simulink model "RobotSystem_2"  (Simulink 5.0)
settings: Solver=ode45  StartTime=0.0  StopTime=SimulationTime  RelTol=1e-3
values from neighbouring files (symbols this model uses):
  d1 = d1 * d1_err    [MakeFourMassRobot.m]
  d2 = d2 * d2_err    [MakeFourMassRobot.m]
  d3 = d3 * d3_err    [MakeFourMassRobot.m]
  DelayTime = DelayTime * DelayTime_err    [MakeFourMassRobot.m]
  fa1 = fa1 * fa1_err    [MakeFourMassRobot.m]
  fa2 = fa2 * fa2_err    [MakeFourMassRobot.m]
  fa3 = fa3 * fa3_err    [MakeFourMassRobot.m]
  FF = 0.50    (= 0.5)    [Controller_1.m]
  fm = fm * fm_err    [MakeFourMassRobot.m]
  Gain = Gain * Gain_err    [MakeFourMassRobot.m]
  gear_ratio = 220    [MakeFourMassRobot.m]
  Ja1 = Ja1 * Ja1_err    [MakeFourMassRobot.m]
  Ja2 = Ja2 * Ja2_err    [MakeFourMassRobot.m]
  Ja3 = Ja3 * Ja3_err    [MakeFourMassRobot.m]
  Jm = Jm * Jm_err    [MakeFourMassRobot.m]
  k1 = k1 * k1_err    [MakeFourMassRobot.m]
  k1_low = k1_low * k1_low_err    [MakeFourMassRobot.m]
  k1_low_pos = 0    [MakeFourMassRobot.m]
  k1_pos = k1_pos * k1_pos_err    [MakeFourMassRobot.m]
  k2 = k2 * k2_err    [MakeFourMassRobot.m]
  k3 = k3 * k3_err    [MakeFourMassRobot.m]
  KD = 1.2    [Controller_1.m]
  KI = 30    [Controller_1.m]
  KP = 12    [Controller_1.m]
  len1 = 20    [MakeFourMassRobot.m]
  len2 = 600    [MakeFourMassRobot.m]
  len3 = 1530    [MakeFourMassRobot.m]
  MotorDisturbance1 = 3.5    [SetParameters.m]
  MotorDisturbance2 = 3.5    [SetParameters.m]
  MotorDisturbance3 = 7    [SetParameters.m]
  MotorDisturbance4 = 4.5    [SetParameters.m]
  MotorDisturbanceChirpAmplitude1 = 1.5    [SetParameters.m]
  MotorDisturbanceChirpAmplitude2 = 1.5    [SetParameters.m]
  MotorDisturbanceChirpEndFrequency1 = 2    [SetParameters.m]
  MotorDisturbanceChirpEndFrequency2 = 2    [SetParameters.m]
  MotorDisturbanceChirpEndTime1 = 21.5    [SetParameters.m]
  MotorDisturbanceChirpEndTime2 = 48    [SetParameters.m]
  MotorDisturbanceChirpStartFrequency1 = 15    [SetParameters.m]
  MotorDisturbanceChirpStartFrequency2 = 15    [SetParameters.m]
  MotorDisturbanceChirpStartTime1 = 16.5    [SetParameters.m]
  MotorDisturbanceChirpStartTime2 = 43    [SetParameters.m]
  MotorDisturbanceOff1 = 5.5    [SetParameters.m]
  MotorDisturbanceOff2 = 25    [SetParameters.m]
  MotorDisturbanceOff3 = 1000    [SetParameters.m]
  MotorDisturbanceOff4 = 32.5    [SetParameters.m]
  MotorDisturbanceOn1 = 5    [SetParameters.m]
  MotorDisturbanceOn2 = 6    [SetParameters.m]
  MotorDisturbanceOn3 = 25    [SetParameters.m]
  MotorDisturbanceOn4 = 32    [SetParameters.m]
  NoiseP = 0.5E-10    (= 5e-11)    [SetParameters.m]
  NoiseTs = 0.5E-3    (= 0.0005)    [SetParameters.m]
  SampleTime = 0.5E-3    (= 0.0005)    [SetParameters.m]
  SimulationTime = 55    [SetParameters.m]
  ToolDisturbance1 = 5    [SetParameters.m]
  ToolDisturbance2 = -7    [SetParameters.m]
  ToolDisturbance3 = 5    [SetParameters.m]
  ToolDisturbanceChirpAmplitude1 = 1.5    [SetParameters.m]
  ToolDisturbanceChirpAmplitude2 = 1.5    [SetParameters.m]
  ToolDisturbanceChirpEndFrequency1 = 2    [SetParameters.m]
  ToolDisturbanceChirpEndFrequency2 = 2    [SetParameters.m]
  ToolDisturbanceChirpEndTime1 = 15.5    [SetParameters.m]
  ToolDisturbanceChirpEndTime2 = 42    [SetParameters.m]
  ToolDisturbanceChirpStartFrequency1 = 15    [SetParameters.m]
  ToolDisturbanceChirpStartFrequency2 = 15    [SetParameters.m]
  ToolDisturbanceChirpStartTime1 = 10.5    [SetParameters.m]
  ToolDisturbanceChirpStartTime2 = 37    [SetParameters.m]
  ToolDisturbanceOff1 = 0.5    [SetParameters.m]
  ToolDisturbanceOff2 = 1000    [SetParameters.m]
  ToolDisturbanceOff3 = 27.5    [SetParameters.m]
  ToolDisturbanceOn1 = 0    [SetParameters.m]
  ToolDisturbanceOn2 = 25    [SetParameters.m]
  ToolDisturbanceOn3 = 27    [SetParameters.m]
  TorqueLimitMax = 20    [SetParameters.m]
  TorqueLimitMin = -20    [SetParameters.m]
libraries: simulink x1
settings Model: LastModifiedBy=STMO  ExtModeTrigMode=oneshot  ExtModeArmWhenConnect=off  LimitDataPoints=off  BlockReductionOpt=off  BooleanDataType=off

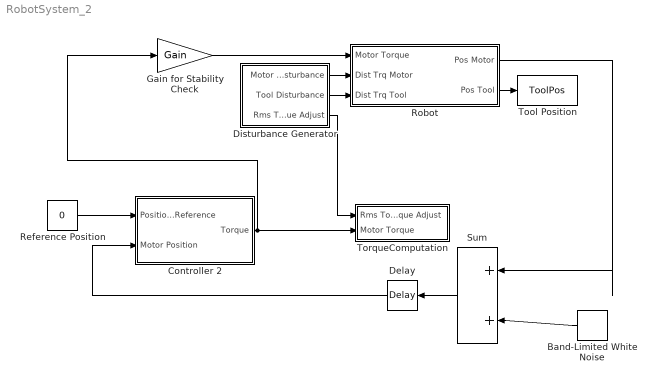
== system RobotSystem_2 ==
  Band-Limited White Noise : simulink/Sources/Band-Limited White Noise  Orientation=left  Cov=[NoiseP]  Ts=NoiseTs  seed=[23341]
  Controller 2 : Subsystem
  Delay : TransportDelay  Orientation=left  DelayTime=DelayTime
  Disturbance Generator : Subsystem
  Gain for Stability Check : Gain  Gain=Gain  SaturateOnIntegerOverflow=on
  Reference Position : Constant  Value=0
  Robot : Subsystem
  Sum : Sum  Orientation=left  Inputs=|++  SaturateOnIntegerOverflow=on
  Tool Position : ToWorkspace  VariableName=ToolPos  SampleTime=-1  SaveFormat=StructureWithTime
  TorqueComputation : Subsystem
  wires:
  Robot/2(Pos Tool) -> Tool Position/1
  Sum/1 -> Delay/1
  Robot/1(Pos Motor) -> Sum/1
  Band-Limited White Noise/1 -> Sum/2
  Disturbance Generator/1(Motor Disturbance) -> Robot/2(Dist Trq Motor)
  Disturbance Generator/2(Tool Disturbance) -> Robot/3(Dist Trq Tool)
  Gain for Stability Check/1 -> Robot/1(Motor Torque)
  Reference Position/1 -> Controller 2/1(Position Reference)
  Delay/1 -> Controller 2/2(Motor Position)
  Controller 2/1(Torque) -> Gain for Stability Check/1, TorqueComputation/2(Motor Torque)
  Disturbance Generator/3(Rms Torque Adjust) -> TorqueComputation/1(Rms Torque Adjust)

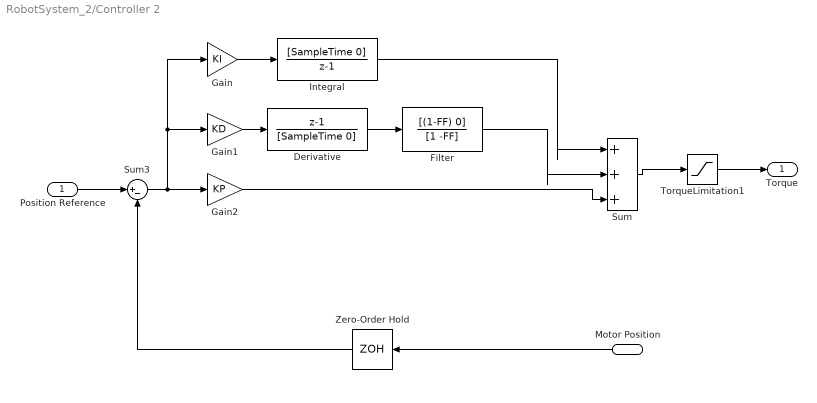
== system RobotSystem_2/Controller 2 ==
  Position Reference : Inport
  Motor Position : Inport  Orientation=left  Port=2
  Derivative : DiscreteTransferFcn  Numerator=[1 -1]  Denominator=[SampleTime 0]  SampleTime=SampleTime
  Filter : DiscreteTransferFcn  Numerator=[(1-FF) 0]  Denominator=[1 -FF]  SampleTime=SampleTime
  Gain : Gain  Gain=KI  SaturateOnIntegerOverflow=on
  Gain1 : Gain  Gain=KD  SaturateOnIntegerOverflow=on
  Gain2 : Gain  Gain=KP  SaturateOnIntegerOverflow=on
  Integral : DiscreteTransferFcn  Numerator=[SampleTime 0]  Denominator=[1 -1]  SampleTime=SampleTime
  Sum : Sum  Inputs=|+++  SaturateOnIntegerOverflow=on
  Sum3 : Sum  Inputs=|+-  SaturateOnIntegerOverflow=on  InputSameDT=on
  TorqueLimitation1 : Saturate  UpperLimit=TorqueLimitMax  LowerLimit=TorqueLimitMin
  Zero-Order Hold : ZeroOrderHold  Orientation=left  SampleTime=SampleTime
  Torque : Outport
  wires:
  Motor Position/1 -> Zero-Order Hold/1
  Position Reference/1 -> Sum3/1
  TorqueLimitation1/1 -> Torque/1
  Zero-Order Hold/1 -> Sum3/2
  Sum/1 -> TorqueLimitation1/1
  Integral/1 -> Sum/1
  Derivative/1 -> Filter/1
  Gain/1 -> Integral/1
  Gain1/1 -> Derivative/1
  Gain2/1 -> Sum/3
  Sum3/1 -> Gain2/1, Gain/1, Gain1/1
  Filter/1 -> Sum/2

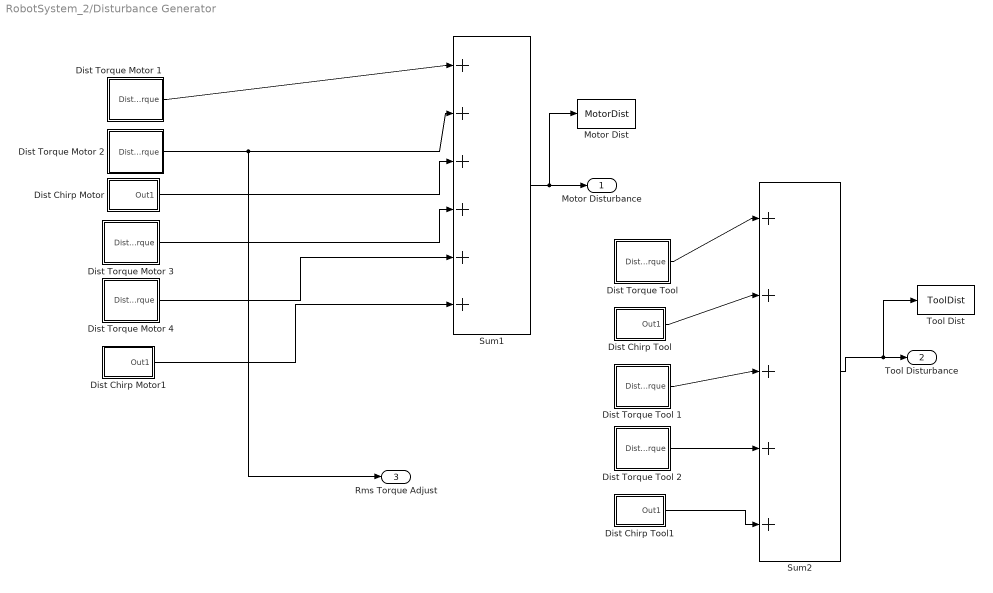
== system RobotSystem_2/Disturbance Generator ==
  Dist Chirp Motor : Subsystem  mask{f1=MotorDisturbanceChirpStartFrequency1, f2=MotorDisturbanceChirpEndFrequency1, T1=MotorDisturbanceChirpStartTime1, T2=MotorDisturbanceChirpEndTime1, Amp=MotorDisturbanceChirpAmplitude1}
      mask prompts: f1 "f1 [Hz]"; f2 "f2 [Hz]"; T1 "T1 [s]"; T2 "T2 [s]"; Amp "Amplitude"
      mask Display: disp('Chirp')
  Dist Chirp Motor1 : Subsystem  mask{f1=MotorDisturbanceChirpStartFrequency2, f2=MotorDisturbanceChirpEndFrequency2, T1=MotorDisturbanceChirpStartTime2, T2=MotorDisturbanceChirpEndTime2, Amp=MotorDisturbanceChirpAmplitude2}
      mask prompts: f1 "f1 [Hz]"; f2 "f2 [Hz]"; T1 "T1 [s]"; T2 "T2 [s]"; Amp "Amplitude"
      mask Display: disp('Chirp')
  Dist Chirp Tool : Subsystem  mask{f1=ToolDisturbanceChirpStartFrequency1, f2=ToolDisturbanceChirpEndFrequency1, T1=ToolDisturbanceChirpStartTime1, T2=ToolDisturbanceChirpEndTime1, Amp=ToolDisturbanceChirpAmplitude1}
      mask prompts: f1 "f1 [Hz]"; f2 "f2 [Hz]"; T1 "T1 [s]"; T2 "T2 [s]"; Amp "Amplitude"
      mask Display: disp('Chirp')
  Dist Chirp Tool1 : Subsystem  mask{f1=ToolDisturbanceChirpStartFrequency2, f2=ToolDisturbanceChirpEndFrequency2, T1=ToolDisturbanceChirpStartTime2, T2=ToolDisturbanceChirpEndTime2, Amp=ToolDisturbanceChirpAmplitude2}
      mask prompts: f1 "f1 [Hz]"; f2 "f2 [Hz]"; T1 "T1 [s]"; T2 "T2 [s]"; Amp "Amplitude"
      mask Display: disp('Chirp')
  Dist Torque Motor 1 : Subsystem  mask{torque=MotorDisturbance1, t1=MotorDisturbanceOn1, t2=MotorDisturbanceOff1}
      mask prompts: torque "Disturbance Torque"; t1 "Pulse On Time"; t2 "Pulse Off Time"
  Dist Torque Motor 2 : Subsystem  mask{torque=MotorDisturbance2, t1=MotorDisturbanceOn2, t2=MotorDisturbanceOff2}
      mask prompts: torque "Disturbance Torque"; t1 "Pulse On Time"; t2 "Pulse Off Time"
  Dist Torque Motor 3 : Subsystem  mask{torque=MotorDisturbance3, t1=MotorDisturbanceOn3, t2=MotorDisturbanceOff3}
      mask prompts: torque "Disturbance Torque"; t1 "Pulse On Time"; t2 "Pulse Off Time"
  Dist Torque Motor 4 : Subsystem  mask{torque=MotorDisturbance4, t1=MotorDisturbanceOn4, t2=MotorDisturbanceOff4}
      mask prompts: torque "Disturbance Torque"; t1 "Pulse On Time"; t2 "Pulse Off Time"
  Dist Torque Tool : Subsystem  mask{torque=ToolDisturbance1, t1=ToolDisturbanceOn1, t2=ToolDisturbanceOff1}
      mask prompts: torque "Disturbance Torque"; t1 "Pulse On Time"; t2 "Pulse Off Time"
  Dist Torque Tool 1 : Subsystem  mask{torque=ToolDisturbance2, t1=ToolDisturbanceOn2, t2=ToolDisturbanceOff2}
      mask prompts: torque "Disturbance Torque"; t1 "Pulse On Time"; t2 "Pulse Off Time"
  Dist Torque Tool 2 : Subsystem  mask{torque=ToolDisturbance3, t1=ToolDisturbanceOn3, t2=ToolDisturbanceOff3}
      mask prompts: torque "Disturbance Torque"; t1 "Pulse On Time"; t2 "Pulse Off Time"
  Motor Dist : ToWorkspace  VariableName=MotorDist  SampleTime=-1  SaveFormat=StructureWithTime
  Sum1 : Sum  Inputs=|++++++  SaturateOnIntegerOverflow=on  InputSameDT=on
  Sum2 : Sum  Inputs=|+++++  SaturateOnIntegerOverflow=on  InputSameDT=on
  Tool Dist : ToWorkspace  VariableName=ToolDist  SampleTime=-1  SaveFormat=StructureWithTime
  Motor Disturbance : Outport
  Tool Disturbance : Outport  Port=2
  Rms Torque Adjust : Outport  Port=3
  wires:
  Dist Torque Motor 1/1(Dist Torque) -> Sum1/1
  Dist Torque Tool/1(Dist Torque) -> Sum2/1
  Dist Chirp Motor/1(Out1) -> Sum1/3
  Dist Chirp Tool/1(Out1) -> Sum2/2
  Sum1/1 -> Motor Dist/1, Motor Disturbance/1
  Sum2/1 -> Tool Disturbance/1, Tool Dist/1
  Dist Torque Motor 3/1(Dist Torque) -> Sum1/4
  Dist Torque Motor 2/1(Dist Torque) -> Sum1/2, Rms Torque Adjust/1
  Dist Torque Tool 1/1(Dist Torque) -> Sum2/3
  Dist Torque Motor 4/1(Dist Torque) -> Sum1/5
  Dist Chirp Motor1/1(Out1) -> Sum1/6
  Dist Chirp Tool1/1(Out1) -> Sum2/5
  Dist Torque Tool 2/1(Dist Torque) -> Sum2/4

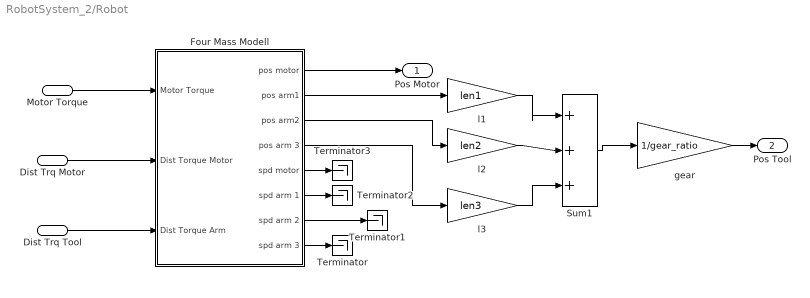
== system RobotSystem_2/Robot ==
  Motor Torque : Inport
  Dist Trq Motor : Inport  Port=2
  Dist Trq Tool : Inport  Port=3
  Four Mass Modell : Subsystem
  Sum1 : Sum  Inputs=|+++  SaturateOnIntegerOverflow=on  InputSameDT=on
  Terminator{,1..3} (4 alike) : Terminator
  gear : Gain  Gain=1/gear_ratio  SaturateOnIntegerOverflow=on
  l1 : Gain  Gain=len1  SaturateOnIntegerOverflow=on
  l2 : Gain  Gain=len2  SaturateOnIntegerOverflow=on
  l3 : Gain  Gain=len3  SaturateOnIntegerOverflow=on
  Pos Motor : Outport
  Pos Tool : Outport  Port=2
  wires:
  Motor Torque/1 -> Four Mass Modell/1(Motor Torque)
  Dist Trq Tool/1 -> Four Mass Modell/3(Dist Torque Arm)
  Dist Trq Motor/1 -> Four Mass Modell/2(Dist Torque Motor)
  Four Mass Modell/1(pos motor) -> Pos Motor/1
  Four Mass Modell/8(spd arm 3) -> Terminator/1
  Four Mass Modell/7(spd arm 2) -> Terminator1/1
  Four Mass Modell/6(spd arm 1) -> Terminator2/1
  Four Mass Modell/5(spd motor) -> Terminator3/1
  Four Mass Modell/3(pos arm2) -> l2/1
  Four Mass Modell/2(pos arm1) -> l1/1
  Four Mass Modell/4(pos arm 3) -> l3/1
  l1/1 -> Sum1/1
  l2/1 -> Sum1/2
  l3/1 -> Sum1/3
  gear/1 -> Pos Tool/1
  Sum1/1 -> gear/1

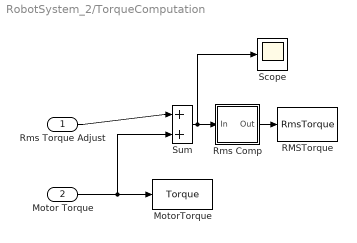
== system RobotSystem_2/TorqueComputation ==
  Rms Torque Adjust : Inport
  Motor Torque : Inport  Port=2
  MotorTorque : ToWorkspace  VariableName=Torque  SampleTime=-1  SaveFormat=StructureWithTime
  RMSTorque : ToWorkspace  VariableName=RmsTorque  SampleTime=-1  SaveFormat=StructureWithTime
  Rms Comp : Subsystem
  Scope : Scope
  Sum : Sum  Inputs=|++  SaturateOnIntegerOverflow=on
  wires:
  Rms Comp/1(Out) -> RMSTorque/1
  Sum/1 -> Rms Comp/1(In), Scope/1
  Rms Torque Adjust/1 -> Sum/1
  Motor Torque/1 -> Sum/2, MotorTorque/1

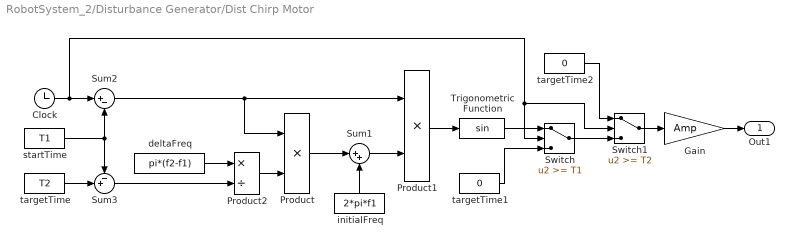
== system RobotSystem_2/Disturbance Generator/Dist Chirp Motor ==
  Clock : Clock
      settings: Decimation=10
  Gain : Gain  Gain=Amp  SaturateOnIntegerOverflow=on
  Product : Product  SaturateOnIntegerOverflow=on  InputSameDT=on
  Product1 : Product  SaturateOnIntegerOverflow=on  InputSameDT=on
  Product2 : Product  Inputs=*/  SaturateOnIntegerOverflow=on  InputSameDT=on
  Sum1 : Sum  Inputs=|++  SaturateOnIntegerOverflow=on  InputSameDT=on
  Sum2 : Sum  Inputs=|+-  SaturateOnIntegerOverflow=on  InputSameDT=on
  Sum3 : Sum  Inputs=-+|  SaturateOnIntegerOverflow=on  InputSameDT=on
  Switch : Switch  Threshold=T1  SaturateOnIntegerOverflow=on  InputSameDT=on
  Switch1 : Switch  Threshold=T2  SaturateOnIntegerOverflow=on  InputSameDT=on
  Trigonometric Function : Trigonometry
  deltaFreq : Constant  Value=pi*(f2-f1)
  initialFreq : Constant  Orientation=up  Value=2*pi*f1
  startTime : Constant  Value=T1
  targetTime : Constant  Value=T2
  targetTime1 : Constant  Value=0
  targetTime2 : Constant  Value=0
  Out1 : Outport
  wires:
  startTime/1 -> Sum3/1, Sum2/2
  Sum2/1 -> Product/1, Product1/1
  Product1/1 -> Trigonometric Function/1
  Sum1/1 -> Product1/2
  Sum3/1 -> Product2/2
  deltaFreq/1 -> Product2/1
  Product2/1 -> Product/2
  targetTime/1 -> Sum3/2
  Clock/1 -> Sum2/1, Switch/2, Switch1/2
  initialFreq/1 -> Sum1/2
  Product/1 -> Sum1/1
  Trigonometric Function/1 -> Switch/1
  targetTime1/1 -> Switch/3
  Switch/1 -> Switch1/3
  Switch1/1 -> Gain/1
  targetTime2/1 -> Switch1/1
  Gain/1 -> Out1/1

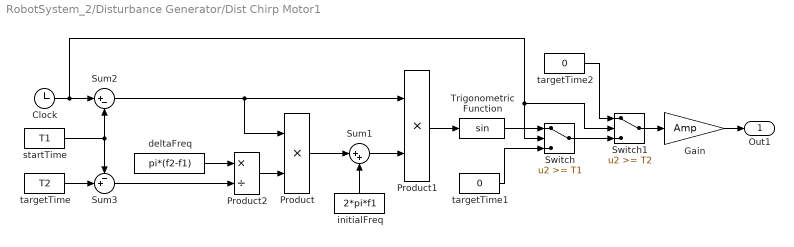
== system RobotSystem_2/Disturbance Generator/Dist Chirp Motor1 ==
  Clock : Clock
      settings: Decimation=10
  Gain : Gain  Gain=Amp  SaturateOnIntegerOverflow=on
  Product : Product  SaturateOnIntegerOverflow=on  InputSameDT=on
  Product1 : Product  SaturateOnIntegerOverflow=on  InputSameDT=on
  Product2 : Product  Inputs=*/  SaturateOnIntegerOverflow=on  InputSameDT=on
  Sum1 : Sum  Inputs=|++  SaturateOnIntegerOverflow=on  InputSameDT=on
  Sum2 : Sum  Inputs=|+-  SaturateOnIntegerOverflow=on  InputSameDT=on
  Sum3 : Sum  Inputs=-+|  SaturateOnIntegerOverflow=on  InputSameDT=on
  Switch : Switch  Threshold=T1  SaturateOnIntegerOverflow=on  InputSameDT=on
  Switch1 : Switch  Threshold=T2  SaturateOnIntegerOverflow=on  InputSameDT=on
  Trigonometric Function : Trigonometry
  deltaFreq : Constant  Value=pi*(f2-f1)
  initialFreq : Constant  Orientation=up  Value=2*pi*f1
  startTime : Constant  Value=T1
  targetTime : Constant  Value=T2
  targetTime1 : Constant  Value=0
  targetTime2 : Constant  Value=0
  Out1 : Outport
  wires:
  startTime/1 -> Sum3/1, Sum2/2
  Sum2/1 -> Product/1, Product1/1
  Product1/1 -> Trigonometric Function/1
  Sum1/1 -> Product1/2
  Sum3/1 -> Product2/2
  deltaFreq/1 -> Product2/1
  Product2/1 -> Product/2
  targetTime/1 -> Sum3/2
  Clock/1 -> Sum2/1, Switch/2, Switch1/2
  initialFreq/1 -> Sum1/2
  Product/1 -> Sum1/1
  Trigonometric Function/1 -> Switch/1
  targetTime1/1 -> Switch/3
  Switch/1 -> Switch1/3
  Switch1/1 -> Gain/1
  targetTime2/1 -> Switch1/1
  Gain/1 -> Out1/1

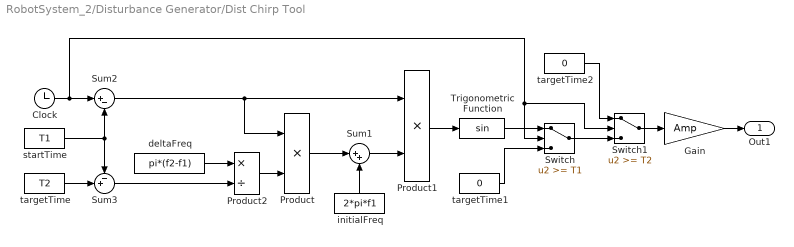
== system RobotSystem_2/Disturbance Generator/Dist Chirp Tool ==
  Clock : Clock
      settings: Decimation=10
  Gain : Gain  Gain=Amp  SaturateOnIntegerOverflow=on
  Product : Product  SaturateOnIntegerOverflow=on  InputSameDT=on
  Product1 : Product  SaturateOnIntegerOverflow=on  InputSameDT=on
  Product2 : Product  Inputs=*/  SaturateOnIntegerOverflow=on  InputSameDT=on
  Sum1 : Sum  Inputs=|++  SaturateOnIntegerOverflow=on  InputSameDT=on
  Sum2 : Sum  Inputs=|+-  SaturateOnIntegerOverflow=on  InputSameDT=on
  Sum3 : Sum  Inputs=-+|  SaturateOnIntegerOverflow=on  InputSameDT=on
  Switch : Switch  Threshold=T1  SaturateOnIntegerOverflow=on  InputSameDT=on
  Switch1 : Switch  Threshold=T2  SaturateOnIntegerOverflow=on  InputSameDT=on
  Trigonometric Function : Trigonometry
  deltaFreq : Constant  Value=pi*(f2-f1)
  initialFreq : Constant  Orientation=up  Value=2*pi*f1
  startTime : Constant  Value=T1
  targetTime : Constant  Value=T2
  targetTime1 : Constant  Value=0
  targetTime2 : Constant  Value=0
  Out1 : Outport
  wires:
  startTime/1 -> Sum3/1, Sum2/2
  Sum2/1 -> Product/1, Product1/1
  Product1/1 -> Trigonometric Function/1
  Sum1/1 -> Product1/2
  Sum3/1 -> Product2/2
  deltaFreq/1 -> Product2/1
  Product2/1 -> Product/2
  targetTime/1 -> Sum3/2
  Clock/1 -> Sum2/1, Switch/2, Switch1/2
  initialFreq/1 -> Sum1/2
  Product/1 -> Sum1/1
  Trigonometric Function/1 -> Switch/1
  targetTime1/1 -> Switch/3
  Switch/1 -> Switch1/3
  Switch1/1 -> Gain/1
  targetTime2/1 -> Switch1/1
  Gain/1 -> Out1/1

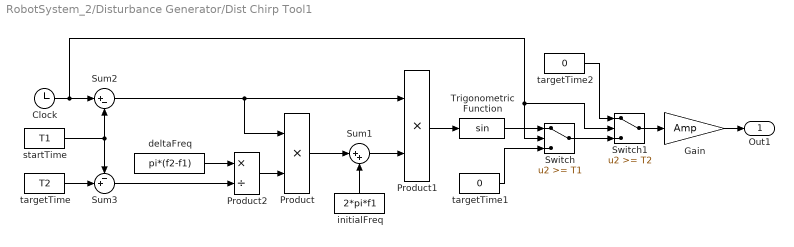
== system RobotSystem_2/Disturbance Generator/Dist Chirp Tool1 ==
  Clock : Clock
      settings: Decimation=10
  Gain : Gain  Gain=Amp  SaturateOnIntegerOverflow=on
  Product : Product  SaturateOnIntegerOverflow=on  InputSameDT=on
  Product1 : Product  SaturateOnIntegerOverflow=on  InputSameDT=on
  Product2 : Product  Inputs=*/  SaturateOnIntegerOverflow=on  InputSameDT=on
  Sum1 : Sum  Inputs=|++  SaturateOnIntegerOverflow=on  InputSameDT=on
  Sum2 : Sum  Inputs=|+-  SaturateOnIntegerOverflow=on  InputSameDT=on
  Sum3 : Sum  Inputs=-+|  SaturateOnIntegerOverflow=on  InputSameDT=on
  Switch : Switch  Threshold=T1  SaturateOnIntegerOverflow=on  InputSameDT=on
  Switch1 : Switch  Threshold=T2  SaturateOnIntegerOverflow=on  InputSameDT=on
  Trigonometric Function : Trigonometry
  deltaFreq : Constant  Value=pi*(f2-f1)
  initialFreq : Constant  Orientation=up  Value=2*pi*f1
  startTime : Constant  Value=T1
  targetTime : Constant  Value=T2
  targetTime1 : Constant  Value=0
  targetTime2 : Constant  Value=0
  Out1 : Outport
  wires:
  startTime/1 -> Sum3/1, Sum2/2
  Sum2/1 -> Product/1, Product1/1
  Product1/1 -> Trigonometric Function/1
  Sum1/1 -> Product1/2
  Sum3/1 -> Product2/2
  deltaFreq/1 -> Product2/1
  Product2/1 -> Product/2
  targetTime/1 -> Sum3/2
  Clock/1 -> Sum2/1, Switch/2, Switch1/2
  initialFreq/1 -> Sum1/2
  Product/1 -> Sum1/1
  Trigonometric Function/1 -> Switch/1
  targetTime1/1 -> Switch/3
  Switch/1 -> Switch1/3
  Switch1/1 -> Gain/1
  targetTime2/1 -> Switch1/1
  Gain/1 -> Out1/1

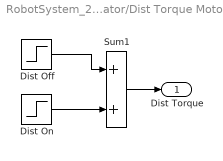
== system RobotSystem_2/Disturbance Generator/Dist Torque Motor 1 ==
  Dist Off : Step  Time=t2  After=-torque  SampleTime=0
  Dist On : Step  Time=t1  After=torque  SampleTime=0
  Sum1 : Sum  Inputs=|++  SaturateOnIntegerOverflow=on  InputSameDT=on
  Dist Torque : Outport
  wires:
  Dist On/1 -> Sum1/2
  Dist Off/1 -> Sum1/1
  Sum1/1 -> Dist Torque/1

== system RobotSystem_2/Disturbance Generator/Dist Torque Motor 2 ==
  Dist Off : Step  Time=t2  After=-torque  SampleTime=0
  Dist On : Step  Time=t1  After=torque  SampleTime=0
  Sum1 : Sum  Inputs=|++  SaturateOnIntegerOverflow=on  InputSameDT=on
  Dist Torque : Outport
  wires:
  Dist On/1 -> Sum1/2
  Dist Off/1 -> Sum1/1
  Sum1/1 -> Dist Torque/1

== system RobotSystem_2/Disturbance Generator/Dist Torque Motor 3 ==
  Dist Off : Step  Time=t2  After=-torque  SampleTime=0
  Dist On : Step  Time=t1  After=torque  SampleTime=0
  Sum1 : Sum  Inputs=|++  SaturateOnIntegerOverflow=on  InputSameDT=on
  Dist Torque : Outport
  wires:
  Dist On/1 -> Sum1/2
  Dist Off/1 -> Sum1/1
  Sum1/1 -> Dist Torque/1

== system RobotSystem_2/Disturbance Generator/Dist Torque Motor 4 ==
  Dist Off : Step  Time=t2  After=-torque  SampleTime=0
  Dist On : Step  Time=t1  After=torque  SampleTime=0
  Sum1 : Sum  Inputs=|++  SaturateOnIntegerOverflow=on  InputSameDT=on
  Dist Torque : Outport
  wires:
  Dist On/1 -> Sum1/2
  Dist Off/1 -> Sum1/1
  Sum1/1 -> Dist Torque/1

== system RobotSystem_2/Disturbance Generator/Dist Torque Tool ==
  Dist Off : Step  Time=t2  After=-torque  SampleTime=0
  Dist On : Step  Time=t1  After=torque  SampleTime=0
  Sum1 : Sum  Inputs=|++  SaturateOnIntegerOverflow=on  InputSameDT=on
  Dist Torque : Outport
  wires:
  Dist On/1 -> Sum1/2
  Dist Off/1 -> Sum1/1
  Sum1/1 -> Dist Torque/1

== system RobotSystem_2/Disturbance Generator/Dist Torque Tool 1 ==
  Dist Off : Step  Time=t2  After=-torque  SampleTime=0
  Dist On : Step  Time=t1  After=torque  SampleTime=0
  Sum1 : Sum  Inputs=|++  SaturateOnIntegerOverflow=on  InputSameDT=on
  Dist Torque : Outport
  wires:
  Dist On/1 -> Sum1/2
  Dist Off/1 -> Sum1/1
  Sum1/1 -> Dist Torque/1

== system RobotSystem_2/Disturbance Generator/Dist Torque Tool 2 ==
  Dist Off : Step  Time=t2  After=-torque  SampleTime=0
  Dist On : Step  Time=t1  After=torque  SampleTime=0
  Sum1 : Sum  Inputs=|++  SaturateOnIntegerOverflow=on  InputSameDT=on
  Dist Torque : Outport
  wires:
  Dist On/1 -> Sum1/2
  Dist Off/1 -> Sum1/1
  Sum1/1 -> Dist Torque/1

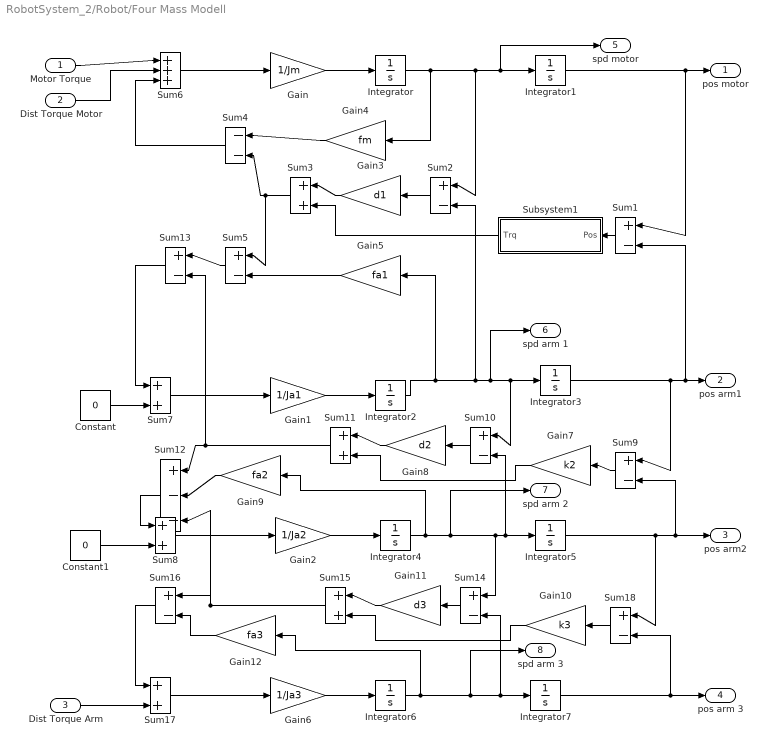
== system RobotSystem_2/Robot/Four Mass Modell ==
  Motor Torque : Inport
  Dist Torque Motor : Inport  Port=2
  Dist Torque Arm : Inport  Port=3
  Constant : Constant  Value=0
  Constant1 : Constant  Value=0
  Gain : Gain  Gain=1/Jm  SaturateOnIntegerOverflow=on
  Gain1 : Gain  Gain=1/Ja1  SaturateOnIntegerOverflow=on
  Gain10 : Gain  Orientation=left  Gain=k3  SaturateOnIntegerOverflow=on
  Gain11 : Gain  Orientation=left  Gain=d3  SaturateOnIntegerOverflow=on
  Gain12 : Gain  Orientation=left  Gain=fa3  SaturateOnIntegerOverflow=on
  Gain2 : Gain  Gain=1/Ja2  SaturateOnIntegerOverflow=on
  Gain3 : Gain  Orientation=left  Gain=d1  SaturateOnIntegerOverflow=on
  Gain4 : Gain  Orientation=left  Gain=fm  SaturateOnIntegerOverflow=on
  Gain5 : Gain  Orientation=left  Gain=fa1  SaturateOnIntegerOverflow=on
  Gain6 : Gain  Gain=1/Ja3  SaturateOnIntegerOverflow=on
  Gain7 : Gain  Orientation=left  Gain=k2  SaturateOnIntegerOverflow=on
  Gain8 : Gain  Orientation=left  Gain=d2  SaturateOnIntegerOverflow=on
  Gain9 : Gain  Orientation=left  Gain=fa2  SaturateOnIntegerOverflow=on
  Integrator{,1..7} (8 alike) : Integrator
  Subsystem1 : Subsystem  Orientation=left  mask{dp1=k1_low_pos, k1=k1_low, dp2=k1_pos, k2=k1, gl=0.0, scale=gear_ratio/60/180*pi}
      mask prompts: dp1 "Dphi1 [bm arm side]"; k1 "Stiffness at dphi1"; dp2 "Dphi2 [bm arm side]"; k2 "Stiffness at dphi2"; gl "Backlash (bm on arm side)"; scale "Scale (n/60/180*pi if dphi & backlash in [bm arm])"
      mask init:
      | dp1=dp1*scale;
      | dp2=dp2*scale;
      | gl=gl*scale;
      | dx=(dp2-dp1)/4;
      | dk=(k2-k1)/4;
      | x1=gl/2;
      | x2=x1+dx;
      | x3=x2+dx;
      | x4=x3+dx;
      | x5=x4+dx;
      | x6=x5+dx;
      | y1=0;
      | y2=y1+dx*k1;
      | y3=y2+dx*(k1+dk);
      | y4=y3+dx*(k1+2*dk);
      | y5=y4+dx*(k1+3*dk);
      | y6=y5+dx*(k1+4*dk);
      mask Display: disp('Nonlinear Spring')
  Sum{1..2,5,9..10,13..14,16,18} (9 alike) : Sum  Orientation=left  Inputs=|+-  SaturateOnIntegerOverflow=on  InputSameDT=on
  Sum11 : Sum  Orientation=left  Inputs=|++  SaturateOnIntegerOverflow=on  InputSameDT=on
  Sum12 : Sum  Orientation=left  Inputs=|+--  SaturateOnIntegerOverflow=on  InputSameDT=on
  Sum15 : Sum  Orientation=left  Inputs=|++  SaturateOnIntegerOverflow=on  InputSameDT=on
  Sum17 : Sum  Inputs=|++  SaturateOnIntegerOverflow=on  InputSameDT=on
  Sum3 : Sum  Orientation=left  Inputs=|++  SaturateOnIntegerOverflow=on  InputSameDT=on
  Sum4 : Sum  Orientation=left  Inputs=|--  SaturateOnIntegerOverflow=on  InputSameDT=on
  Sum6 : Sum  Inputs=|+++  SaturateOnIntegerOverflow=on  InputSameDT=on
  Sum7 : Sum  Inputs=|++  SaturateOnIntegerOverflow=on  InputSameDT=on
  Sum8 : Sum  Inputs=|++  SaturateOnIntegerOverflow=on  InputSameDT=on
  pos motor : Outport
  pos arm1 : Outport  Port=2
  pos arm2 : Outport  Port=3
  pos arm 3 : Outport  Port=4
  spd motor : Outport  Port=5
  spd arm 1 : Outport  Port=6
  spd arm 2 : Outport  Port=7
  spd arm 3 : Outport  Port=8
  wires:
  Gain/1 -> Integrator/1
  Sum6/1 -> Gain/1
  Motor Torque/1 -> Sum6/1
  Integrator1/1 -> Sum1/1, pos motor/1
  Gain4/1 -> Sum4/1
  Integrator/1 -> Sum2/1, Integrator1/1, spd motor/1, Gain4/1
  Gain2/1 -> Integrator4/1
  Gain1/1 -> Integrator2/1
  Sum2/1 -> Gain3/1
  Integrator2/1 -> Sum2/2, Integrator3/1, Sum10/1, spd arm 1/1, Gain5/1
  Gain3/1 -> Sum3/1
  Gain5/1 -> Sum5/2
  Sum3/1 -> Sum4/2, Sum5/1
  Sum7/1 -> Gain1/1
  Constant/1 -> Sum7/2
  Subsystem1/1(Trq) -> Sum3/2
  Sum1/1 -> Subsystem1/1(Pos)
  Sum8/1 -> Gain2/1
  Constant1/1 -> Sum8/2
  Sum9/1 -> Gain7/1
  Integrator3/1 -> Sum1/2, pos arm1/1, Sum9/1
  Integrator5/1 -> pos arm2/1, Sum9/2, Sum18/1
  Sum10/1 -> Gain8/1
  Gain8/1 -> Sum11/1
  Gain7/1 -> Sum11/2
  Sum12/1 -> Sum8/1
  Gain9/1 -> Sum12/2
  Integrator4/1 -> Gain9/1, Integrator5/1, Sum10/2, Sum14/1, spd arm 2/1
  Sum5/1 -> Sum13/1
  Sum13/1 -> Sum7/1
  Sum11/1 -> Sum12/1, Sum13/2
  Dist Torque Motor/1 -> Sum6/2
  Sum4/1 -> Sum6/3
  Gain6/1 -> Integrator6/1
  Sum17/1 -> Gain6/1
  Dist Torque Arm/1 -> Sum17/2
  Sum18/1 -> Gain10/1
  Integrator7/1 -> pos arm 3/1, Sum18/2
  Sum14/1 -> Gain11/1
  Gain11/1 -> Sum15/1
  Gain10/1 -> Sum15/2
  Sum16/1 -> Sum17/1
  Gain12/1 -> Sum16/2
  Integrator6/1 -> Gain12/1, Integrator7/1, Sum14/2, spd arm 3/1
  Sum15/1 -> Sum16/1, Sum12/3

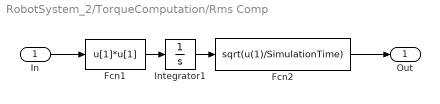
== system RobotSystem_2/TorqueComputation/Rms Comp ==
  In : Inport
  Fcn1 : Fcn  Expr=u[1]*u[1]
  Fcn2 : Fcn  Expr=sqrt(u(1)/SimulationTime)
  Integrator1 : Integrator
  Out : Outport
  wires:
  Fcn1/1 -> Integrator1/1
  In/1 -> Fcn1/1
  Fcn2/1 -> Out/1
  Integrator1/1 -> Fcn2/1

== system RobotSystem_2/Robot/Four Mass Modell/Subsystem1 ==
  Pos : Inport
  Look-Up Table : Lookup  InputValues=[-x6 -x5 -x4 -x3 -x2 -x1 0 x1 x2 x3 x4 x5 x6]  OutputValues=[-y6 -y5 -y4 -y3 -y2 0 0 0 y2 y3 y4 y5 y6]  SaturateOnIntegerOverflow=on
  Trq : Outport
  wires:
  Look-Up Table/1 -> Trq/1
  Pos/1 -> Look-Up Table/1
